simulink model "longitudinal_model"  (R2019b)
settings: Solver=VariableStepAuto  StartTime=0.0  StopTime=10.0  RelTol=1e-3
values from neighbouring files (symbols this model uses):
  airDensity = 1.225    [longitudinalModel.m]
  Cd = 0.3    [longitudinalModel.m]
  distanceCGAxleFront = 1    [longitudinalModel.m]
  distanceCGAxleRear = 1    [longitudinalModel.m]
  frontalArea = 0.7    [longitudinalModel.m]
  gravity = 9.8    [longitudinalModel.m]
  heightCG = 0.4    [longitudinalModel.m]
  massVehicle = 329    [longitudinalModel.m]
  momentInertia = 0.7    [longitudinalModel.m]
  radiusWheel = 0.25    [longitudinalModel.m]
  SR = [-0.15	-0.14	-0.13	-0.12	-0.11	-0.1	-0.09	-0.08	-0.07	-0.06	-0.05	-0.04	-0.03	-0.02	-0.01	0	0.01	0.02	0.03	0.04	0.05	0.06	0.07	0.08	0.09	0.1	0.11	0.12	0.13	0.14	0.15]    [longitudinalModel.m]
  sumDistanceCGAxles = distanceCGAxleRear + distanceCGAxleFront    (= 2)    [longitudinalModel.m]
settings Model: SimulationMode=rapid-accelerator  Creator=Helen Ikeda  LastModifiedBy=Helen Ikeda

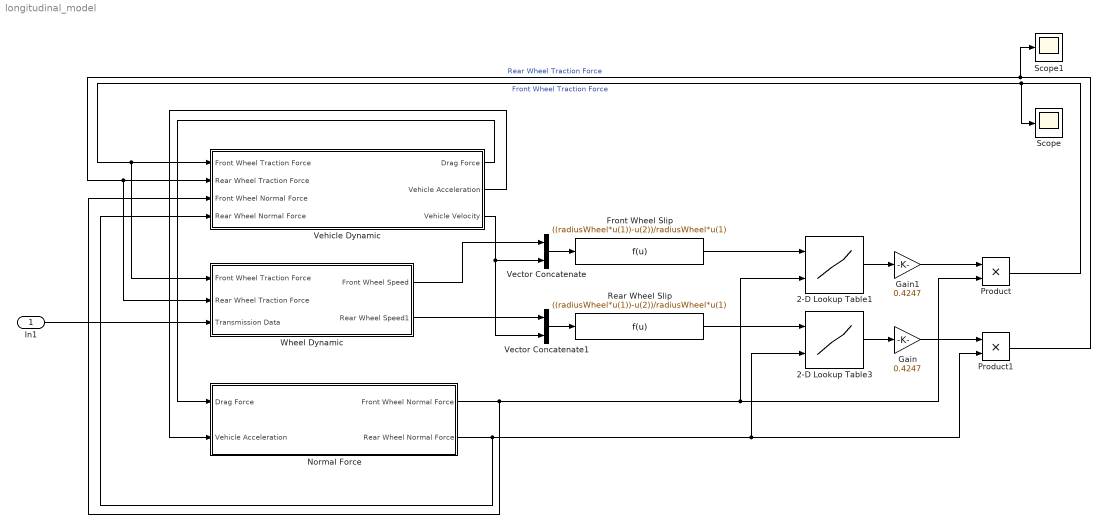
== system longitudinal_model ==
  In1 : Inport
  2-D Lookup Table1 : Lookup_n-D  BreakpointsForDimension1=SR  BreakpointsForDimension2=load  Table=u  InternalRulePriority=Speed  OutDataTypeStr=Inherit: Inherit from 'Table data'  RndMeth=Simplest  InputSameDT=on
  2-D Lookup Table3 : Lookup_n-D  BreakpointsForDimension1=SR  BreakpointsForDimension2=load  Table=u  InternalRulePriority=Speed  OutDataTypeStr=Inherit: Inherit from 'Table data'  RndMeth=Simplest  InputSameDT=on
  Front Wheel Slip : Fcn  Expr=((radiusWheel*u(1))-u(2))/radiusWheel*u(1)
  Gain : Gain  Gain=0.4247
  Gain1 : Gain  Gain=0.4247
  "Normal Force " : Subsystem
  Product : Product
  Product1 : Product
  Rear Wheel Slip : Fcn  Expr=((radiusWheel*u(1))-u(2))/radiusWheel*u(1)
  Scope : Scope
  Scope1 : Scope
  Vector Concatenate : Concatenate
  Vector Concatenate1 : Concatenate
  Vehicle Dynamic : Subsystem
  Wheel Dynamic : Subsystem
  wires:
  Vehicle Dynamic/2(Vehicle Acceleration) -> "Normal Force "/2(Vehicle Acceleration)
  Vehicle Dynamic/1(Drag Force) -> "Normal Force "/1(Drag Force)
  Vector Concatenate/1 -> Front Wheel Slip/1
  Vector Concatenate1/1 -> Rear Wheel Slip/1
  Wheel Dynamic/1(Front Wheel Speed) -> Vector Concatenate/1
  Vehicle Dynamic/3(Vehicle Velocity) -> Vector Concatenate1/2, Vector Concatenate/2
  Wheel Dynamic/2(Rear Wheel Speed1) -> Vector Concatenate1/1
  "Normal Force "/1(Front Wheel Normal Force) -> Product/2, 2-D Lookup Table1/2, Vehicle Dynamic/3(Front Wheel Normal Force)
  "Normal Force "/2(Rear Wheel Normal Force) -> Vehicle Dynamic/4(Rear Wheel Normal Force), 2-D Lookup Table3/2, Product1/2
  Product/1 -> Scope/1, Wheel Dynamic/1(Front Wheel Traction Force), Vehicle Dynamic/1(Front Wheel Traction Force)  "Front Wheel Traction Force"
  Product1/1 -> Scope1/1, Wheel Dynamic/2(Rear Wheel Traction Force), Vehicle Dynamic/2(Rear Wheel Traction Force)  "Rear Wheel Traction Force"
  In1/1 -> Wheel Dynamic/3(Transmission Data)
  2-D Lookup Table3/1 -> Gain/1
  Rear Wheel Slip/1 -> 2-D Lookup Table3/1
  Gain/1 -> Product1/1
  2-D Lookup Table1/1 -> Gain1/1
  Front Wheel Slip/1 -> 2-D Lookup Table1/1
  Gain1/1 -> Product/1

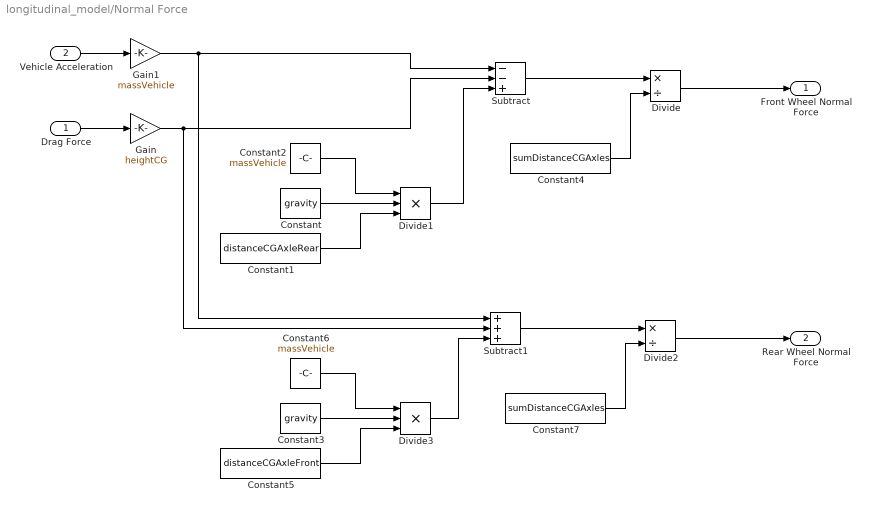
== system longitudinal_model/Normal Force  ==
  Drag Force : Inport
  Vehicle Acceleration : Inport  Port=2
  Constant : Constant  Value=gravity
  Constant1 : Constant  Value=distanceCGAxleRear
  Constant2 : Constant  Value=massVehicle
  Constant3 : Constant  Value=gravity
  Constant4 : Constant  Value=sumDistanceCGAxles
  Constant5 : Constant  Value=distanceCGAxleFront
  Constant6 : Constant  Value=massVehicle
  Constant7 : Constant  Value=sumDistanceCGAxles
  Divide : Product  Inputs=*/
  Divide1 : Product  Inputs=***
  Divide2 : Product  Inputs=*/
  Divide3 : Product  Inputs=***
  Gain : Gain  Gain=heightCG
  Gain1 : Gain  Gain=massVehicle
  Subtract : Sum  Inputs=--+
  Subtract1 : Sum  Inputs=+++
  Front Wheel Normal Force : Outport
  Rear Wheel Normal Force : Outport  Port=2
  wires:
  Vehicle Acceleration/1 -> Gain1/1
  Drag Force/1 -> Gain/1
  Constant2/1 -> Divide1/1
  Constant/1 -> Divide1/2
  Constant1/1 -> Divide1/3
  Gain1/1 -> Subtract1/1, Subtract/1
  Gain/1 -> Subtract1/2, Subtract/2
  Divide1/1 -> Subtract/3
  Subtract/1 -> Divide/1
  Divide/1 -> Front Wheel Normal Force/1
  Constant4/1 -> Divide/2
  Constant6/1 -> Divide3/1
  Constant7/1 -> Divide2/2
  Constant3/1 -> Divide3/2
  Constant5/1 -> Divide3/3
  Divide3/1 -> Subtract1/3
  Subtract1/1 -> Divide2/1
  Divide2/1 -> Rear Wheel Normal Force/1

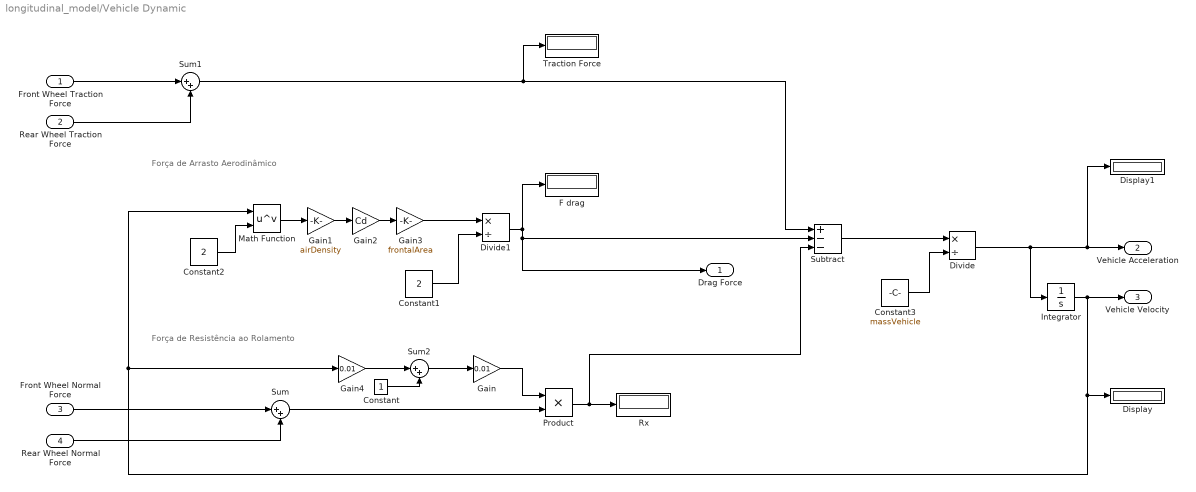
== system longitudinal_model/Vehicle Dynamic ==
  note: Força de Arrasto Aerodinâmico
  note: Força de Resistência ao Rolamento
  Front Wheel Traction Force : Inport
  Rear Wheel Traction Force : Inport  Port=2
  Front Wheel Normal Force : Inport  Port=3
  Rear Wheel Normal Force : Inport  Port=4
  Constant : Constant
  Constant1 : Constant  Value=2
  Constant2 : Constant  Value=2
  Constant3 : Constant  Value=massVehicle
  Display : Display
  Display1 : Display
  Divide : Product  Inputs=*/
  Divide1 : Product  Inputs=*/
  F drag : Display
  Gain : Gain  Gain=0.01
  Gain1 : Gain  Gain=airDensity
  Gain2 : Gain  Gain=Cd
  Gain3 : Gain  Gain=frontalArea
  Gain4 : Gain  Gain=0.01
  Integrator : Integrator
  Math Function : Math  Operator=pow  SignedPower=off  OutputSignalType=real  SaturateOnIntegerOverflow=on
  Product : Product
  "Rx " : Display
  Subtract : Sum  Inputs=+--
  Sum : Sum  Inputs=|++
  Sum1 : Sum  Inputs=|++
  Sum2 : Sum  Inputs=|++
  Traction Force : Display
  Drag Force : Outport
  Vehicle Acceleration : Outport  Port=2
  Vehicle Velocity : Outport  Port=3
  wires:
  Gain3/1 -> Divide1/1
  Constant2/1 -> Math Function/2
  Integrator/1 -> Vehicle Velocity/1, Display/1, Math Function/1, Gain4/1
  Constant1/1 -> Divide1/2
  Math Function/1 -> Gain1/1
  Divide1/1 -> Drag Force/1, Subtract/2, F drag/1
  Subtract/1 -> Divide/1
  Constant3/1 -> Divide/2
  Divide/1 -> Display1/1, Vehicle Acceleration/1, Integrator/1
  Front Wheel Normal Force/1 -> Sum/1
  Rear Wheel Normal Force/1 -> Sum/2
  Front Wheel Traction Force/1 -> Sum1/1
  Rear Wheel Traction Force/1 -> Sum1/2
  Sum1/1 -> Subtract/1, Traction Force/1
  Gain1/1 -> Gain2/1
  Gain2/1 -> Gain3/1
  Gain4/1 -> Sum2/1
  Constant/1 -> Sum2/2
  Sum2/1 -> Gain/1
  Sum/1 -> Product/2
  Gain/1 -> Product/1
  Product/1 -> Subtract/3, "Rx "/1

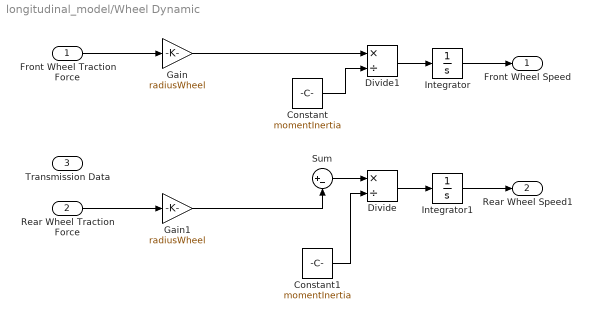
== system longitudinal_model/Wheel Dynamic ==
  Front Wheel Traction Force : Inport
  Rear Wheel Traction Force : Inport  Port=2
  Transmission Data : Inport  Port=3
  Constant : Constant  Value=momentInertia
  Constant1 : Constant  Value=momentInertia
  Divide : Product  Inputs=*/
  Divide1 : Product  Inputs=*/
  Gain : Gain  Gain=radiusWheel
  Gain1 : Gain  Gain=radiusWheel
  Integrator : Integrator
  Integrator1 : Integrator
  Sum : Sum  Inputs=|+-
  Front Wheel Speed : Outport
  Rear Wheel Speed1 : Outport  Port=2
  wires:
  Integrator/1 -> Front Wheel Speed/1
  Integrator1/1 -> Rear Wheel Speed1/1
  Front Wheel Traction Force/1 -> Gain/1
  Rear Wheel Traction Force/1 -> Gain1/1
  Divide/1 -> Integrator1/1
  Gain/1 -> Divide1/1
  Sum/1 -> Divide/1
  Gain1/1 -> Sum/2
  Constant/1 -> Divide1/2
  Constant1/1 -> Divide/2
  Divide1/1 -> Integrator/1
